simulink model "problem_7_model"  (R2020b)
settings: Solver=VariableStepAuto  StartTime=0.0  StopTime=10.0  RelTol=1e-3
libraries: dspsrcs4 x1
settings Model: Creator=gauri  LastModifiedBy=mluser

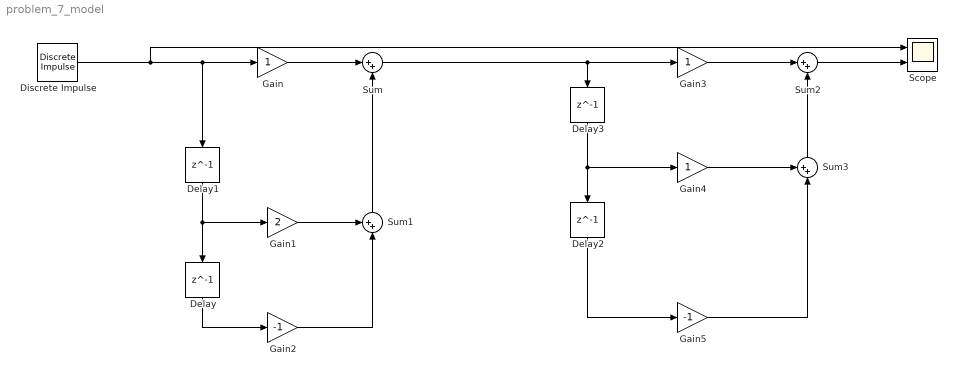
== system problem_7_model ==
  Delay{,1..3} (4 alike) : Delay  DelayLength=1
  Discrete Impulse : dspsrcs4/Discrete  Impulse  Delay=0  SampleTime=1  FrameSample=1  OutputFrames=off  dataType=double  isSigned=on  wordLen=16  udDataType=sfix(16)  fracBitsMode=Best precision  numFracBits=15  OutDataTypeStr=double  LastOutDataTypeStr=double
  Gain : Gain
  Gain1 : Gain  Gain=2
  Gain2 : Gain  Gain=-1
  Gain3 : Gain
  Gain4 : Gain
  Gain5 : Gain  Gain=-1
  Scope : Scope  NumInputPorts=2
  Sum : Sum  Inputs=|++
  Sum1 : Sum  Inputs=++|
  Sum2 : Sum  Inputs=|++
  Sum3 : Sum  Inputs=++|
  wires:
  Delay1/1 -> Gain1/1, Delay/1
  Delay3/1 -> Gain4/1, Delay2/1
  Discrete Impulse/1 -> Scope/1, Gain/1, Delay1/1
  Gain/1 -> Sum/1
  Sum1/1 -> Sum/2
  Gain1/1 -> Sum1/1
  Delay/1 -> Gain2/1
  Gain2/1 -> Sum1/2
  Sum/1 -> Gain3/1, Delay3/1
  Gain3/1 -> Sum2/1
  Sum3/1 -> Sum2/2
  Gain4/1 -> Sum3/1
  Delay2/1 -> Gain5/1
  Gain5/1 -> Sum3/2
  Sum2/1 -> Scope/2
